simulink model "add"  (R2020a)
settings: Solver=VariableStepAuto  StartTime=0.0  StopTime=10.0  RelTol=1e-3
settings Model: Creator=P0158631  LastModifiedBy=P0158631

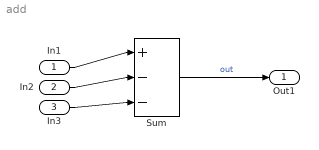
== system add ==
  In1 : Inport
  In2 : Inport  Port=2
  In3 : Inport  Port=3
  Sum : Sum  Inputs=|+--
  Out1 : Outport  SignalName=Out1
  wires:
  Sum/1 -> Out1/1  "out"
  In1/1 -> Sum/1
  In2/1 -> Sum/2
  In3/1 -> Sum/3
